simulink model "inverse_dynamics_control"  (R2019a)
settings: Solver=VariableStepAuto  StartTime=0.0  StopTime=10.0  RelTol=1e-3
undefined symbols (not defined in the file or in its folder): Friction, fwdKine, GravityVector, JacobianDerivative
libraries: robotcorelib x1
settings Model: Creator=shra1  LastModifiedBy=shra1

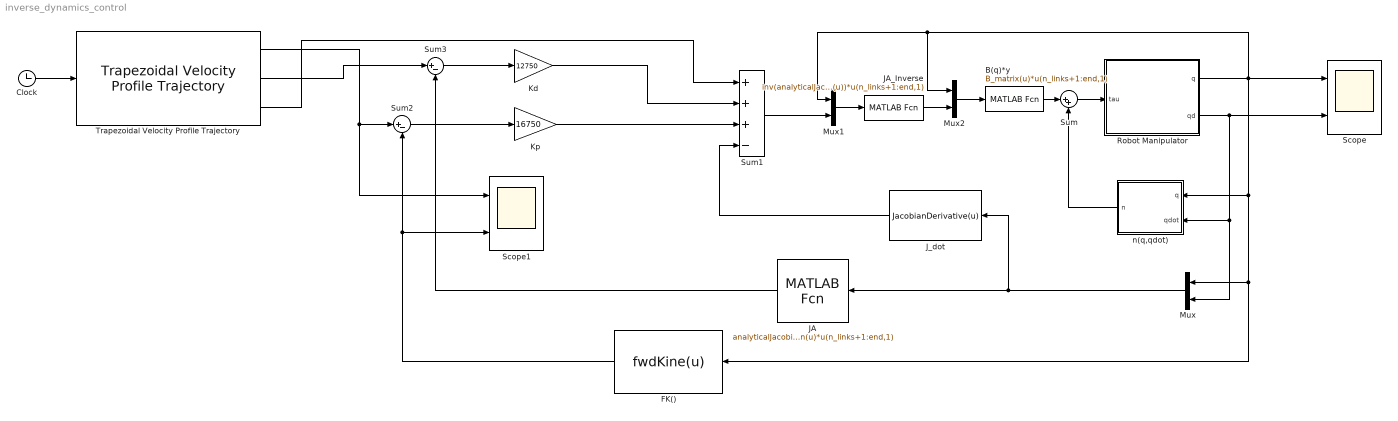
== system inverse_dynamics_control ==
  B(q)*y : MATLABFcn  MATLABFcn=B_matrix(u)*u(n_links+1:end,1)
  Clock : Clock
  FK() : MATLABFcn  MATLABFcn=fwdKine(u)
  JA : MATLABFcn  MATLABFcn=analyticalJacobian(u)*u(n_links+1:end,1)
  JA_Inverse : MATLABFcn  MATLABFcn=inv(analyticalJacobian(u))*u(n_links+1:end,1)
  J_dot : MATLABFcn  MATLABFcn=JacobianDerivative(u)
  Kd : Gain  Gain=12750
  Kp : Gain  Gain=16750
  Mux : Mux  Inputs=2
  Mux1 : Mux  Inputs=2
  Mux2 : Mux  Inputs=2
  Robot Manipulator : Subsystem
  Scope : Scope  NumInputPorts=2
  Scope1 : Scope  NumInputPorts=2
  Sum : Sum  Inputs=|++
  Sum1 : Sum  Inputs=+++-  SaturateOnIntegerOverflow=on  InputSameDT=on  OutDataTypeStr=Inherit: Same as first input
  Sum2 : Sum  Inputs=|+-
  Sum3 : Sum  Inputs=|+-
  Trapezoidal Velocity Profile Trajectory : robotcorelib/Trapezoidal Velocity Profile Trajectory  WaypointSource=Internal  Waypoints=[0.2018, 0.59; 0.6832, 0.4631; 0,0]  NumParams=0  Parameter1=Peak Velocity  Parameter2=End Time  ParameterSource=Internal  PeakVelocity=[ 2; 2 ]  Acceleration=[ 1; 2 ]  EndTime=[ 1; 1 ]  AccelTime=[ 1; 2 ]  SimulateUsing=Interpreted execution
      settings: SourceProductName=Robotics System Toolbox  SourceProductBaseCode=RO
  n(q,qdot) : Subsystem
  wires:
  Sum2/1 -> Kp/1
  Sum/1 -> Robot Manipulator/1(tau)
  Kp/1 -> Sum1/3
  Trapezoidal Velocity Profile Trajectory/1 -> Scope1/1, Sum2/1
  Robot Manipulator/2(qd) -> n(q,qdot)/2(qdot), Mux/2, Scope/2
  FK()/1 -> Scope1/2, Sum2/2
  Mux1/1 -> JA_Inverse/1
  Mux/1 -> J_dot/1, JA/1
  B(q)*y/1 -> Sum/1
  Mux2/1 -> B(q)*y/1
  Robot Manipulator/1(q) -> Mux2/1, Mux1/1, n(q,qdot)/1(q), Mux/1, FK()/1, Scope/1
  JA_Inverse/1 -> Mux2/2
  Sum1/1 -> Mux1/2
  n(q,qdot)/1(n) -> Sum/2
  Sum3/1 -> Kd/1
  JA/1 -> Sum3/2
  Trapezoidal Velocity Profile Trajectory/2 -> Sum3/1
  Kd/1 -> Sum1/2
  J_dot/1 -> Sum1/4
  Trapezoidal Velocity Profile Trajectory/3 -> Sum1/1
  Clock/1 -> Trapezoidal Velocity Profile Trajectory/1

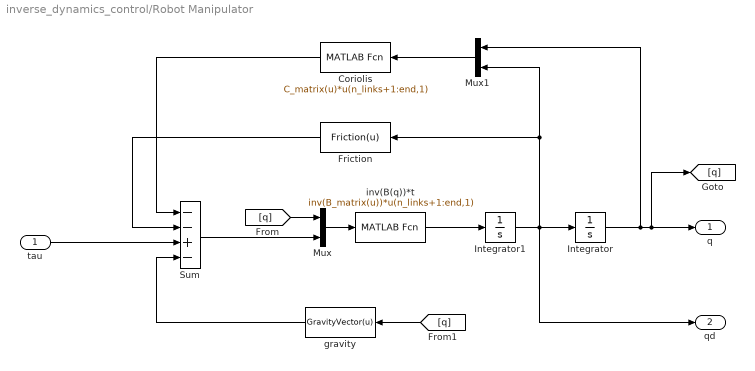
== system inverse_dynamics_control/Robot Manipulator ==
  tau : Inport
  Coriolis : MATLABFcn  MATLABFcn=C_matrix(u)*u(n_links+1:end,1)
  Friction : MATLABFcn  MATLABFcn=Friction(u)
  Integrator : Integrator  InitialCondition=[pi/3; -pi/3 ;0]
  Integrator1 : Integrator  InitialCondition=[0;0;0]
  Mux : Mux  Inputs=2
  Mux1 : Mux  Inputs=2
  Sum : Sum  Inputs=--+-  SaturateOnIntegerOverflow=on  InputSameDT=on  OutDataTypeStr=Inherit: Same as first input
  gravity : MATLABFcn  MATLABFcn=GravityVector(u)
  inv(B(q))*t : MATLABFcn  MATLABFcn=inv(B_matrix(u))*u(n_links+1:end,1)
  q : Outport
  qd : Outport  Port=2
  wires:
  Integrator1/1 -> Friction/1, Mux1/2, qd/1, Integrator/1
  inv(B(q))*t/1 -> Integrator1/1
  Mux/1 -> inv(B(q))*t/1
  [q] -> Mux/1
  Integrator/1 -> Mux1/1, [q], q/1
  tau/1 -> Sum/3
  Mux1/1 -> Coriolis/1
  [q] -> gravity/1
  gravity/1 -> Sum/4
  Coriolis/1 -> Sum/1
  Sum/1 -> Mux/2
  Friction/1 -> Sum/2

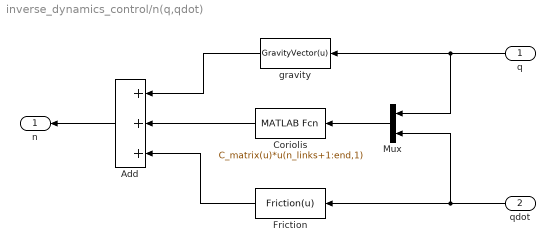
== system inverse_dynamics_control/n(q,qdot) ==
  q : Inport
  qdot : Inport  Port=2
  Add : Sum  Inputs=+++
  Coriolis : MATLABFcn  MATLABFcn=C_matrix(u)*u(n_links+1:end,1)
  Friction : MATLABFcn  MATLABFcn=Friction(u)
  Mux : Mux  Inputs=2
  gravity : MATLABFcn  MATLABFcn=GravityVector(u)
  n : Outport
  wires:
  Coriolis/1 -> Add/2
  gravity/1 -> Add/1
  Friction/1 -> Add/3
  Add/1 -> n/1
  Mux/1 -> Coriolis/1
  q/1 -> Mux/1, gravity/1
  qdot/1 -> Mux/2, Friction/1
